simulink model "FinalCodev2_2"  (R2021b)
settings: Solver=ode23t  StartTime=0.0  StopTime=inf  RelTol=1e-3
InitFcn:
  | RPInit
model workspace (MAT data in the model file):
  mapForSim : object (value not decoded)
  occGrid : robotics.BinaryOccupancyGrid (value not decoded)
undefined symbols (not defined in the file or in its folder): X, Y, Z
libraries: sm_lib x25, nesl_utility x11, RP_Simulator_Components x7, ME598_ProjectLibrary x6, RoboticsPlayground x2, Contact_Forces_Lib x2
(part 2 of 2)

== stateflow chart FinalCodev2_2/Chart ==
  state DriveForward [commented out]
    LMotor = 100
    RMotor = 100
  state PivotRight [commented out]
    LMotor = -100
    RMotor = 100
  state GoToFirstPuck [commented out]
    state DriveForward1 [commented out]
      LeftM = 100;
      RightM = 100;
    state PivotLeft [commented out]
      entry, during:
      theta = atan2d(1.5-y,0-x);
      LeftM = -40;
      RightM = 40;
    state Stop [commented out]
      LeftM = 0;
      RightM = 0;
    (default) -> GoToFirstPuck.PivotLeft [commented out]
    GoToFirstPuck.PivotLeft -> GoToFirstPuck.DriveForward1 [commented out] : [t>theta-5 && t<theta+2]
    GoToFirstPuck.DriveForward1 -> GoToFirstPuck.Stop [commented out] : [Red_Distance < 0.42 && Red_Distance > 0.4]
  state GoToSecondPuck [commented out]
    state DriveForward1 [commented out]
      LeftM = 100;
      RightM = 100;
    state PivotRight [commented out]
      entry, during:
      theta = atan2d(-1.5-y,0-x);
      LeftM = 60;
      RightM = -60;
    state Stop [commented out]
      LeftM = 0;
      RightM = 0;
    (default) -> GoToSecondPuck.PivotRight [commented out]
    GoToSecondPuck.PivotRight -> GoToSecondPuck.DriveForward1 [commented out] : [t>theta-5 && t<theta+2]
    GoToSecondPuck.DriveForward1 -> GoToSecondPuck.Stop [commented out] : [Blue_Distance < 0.42 && Blue_Distance > 0.4]
  state NotCenter [commented out]
    LMotor = 100;
    RMotor = 100;
  state Centered [commented out]
    LMotor = 0;
    RMotor = 0;
  state GoToFirstPuck1
    state PivotLeft
      entry, during:
      theta = atan2d(1.5-y,0-x);
      LeftM = -15;
      RightM = 15;
    state DriveForward1
      entry,during:
      LeftM = 100;
      RightM = 100;
      exit:
      LeftM = 0;
      RightM = 0;
    (default) -> GoToFirstPuck1.PivotLeft
    GoToFirstPuck1.PivotLeft -> GoToFirstPuck1.DriveForward1 : [t>theta-2 && t<theta+2]
  note: NOTES:
      | - Consider a transition loop of pivotleft, pivotright, and moveforward for
      | each larger state blocks.
      | - If the puck is not completely centered on the manipulator, then it will
      | make the robot steer in the direction where the puck is leaning. For
      | example, if the puck is on the left side of the manipulator and you want
      | the robot to move forward, then it will slightly steer to the left. This is
      | unwanted behavior, so it is good to make sure that the theta pose of the
      | robot is always compared to the target pose so the robot doesn't stray from
      | the desired path.
      | - check the closest pivot!
  state GoToFirstEndzone [commented out]
    state PivotRight [commented out]
      entry,during:
      theta = atan2d(2.3-y, 2.3-x);
      LeftM = 40;
      RightM = -40;
    state DriveForward2 [commented out]
      LeftM = 80;
      RightM = 80;
    state Reverse [commented out]
      LeftM = -100;
      RightM = -100;
    state Stop2 [commented out]
      LeftM =0;
      RightM = 0;
    (default) -> GoToFirstEndzone.PivotRight [commented out]
    GoToFirstEndzone.PivotRight -> GoToFirstEndzone.DriveForward2 [commented out] : [t>theta-5 && t< theta+2]
    GoToFirstEndzone.DriveForward2 -> GoToFirstEndzone.Reverse [commented out] : [FrontSensor <0.7]
    GoToFirstEndzone.Reverse -> GoToFirstEndzone.Stop2 [commented out] : after(2,sec)
  state GoToSecondEndzone [commented out]
    state PivotRight [commented out]
      entry,during:
      theta = atan2d(0-y, -2.3-x);
      LeftM = 40;
      RightM = -40;
    state DriveForward2 [commented out]
      LeftM = 80;
      RightM = 80;
    state Reverse [commented out]
      LeftM = -100;
      RightM = -100;
    state Stop2 [commented out]
      LeftM =0;
      RightM = 0;
    (default) -> GoToSecondEndzone.PivotRight [commented out]
    GoToSecondEndzone.PivotRight -> GoToSecondEndzone.DriveForward2 [commented out] : [t>theta-5 && t< theta+2]
    GoToSecondEndzone.DriveForward2 -> GoToSecondEndzone.Reverse [commented out] : [FrontSensor <0.7]
    GoToSecondEndzone.Reverse -> GoToSecondEndzone.Stop2 [commented out] : after(2,sec)
  state GoToRedEndzone
    state PivotRight
      entry,during:
      theta = atan2d(2.2-y, 2.3-x);
      LeftM = 15;
      RightM = -15;
    state DriveForward2
      entry,during:
      theta = atan2d(2.2-y,2.3-x)
      LeftM = 80;
      RightM = 80;
    state Reverse
      entry,during:
      LeftM = -100;
      RightM = -100;
      exit:
      LeftM = 0;
      RightM = 0;
    state LeftWallAvoid
      entry,during:
      LeftM = 80;
      RightM = 0;
    state RightWallAvoid
      entry,during:
      LeftM = 0;
      RightM = 80;
    (default) -> GoToRedEndzone.PivotRight
    GoToRedEndzone.DriveForward2 -> GoToRedEndzone.PivotRight [order 2] : [(t-theta)>0]
    GoToRedEndzone.PivotRight -> GoToRedEndzone.DriveForward2 : [t>theta-2 && t< theta+2]
    GoToRedEndzone.DriveForward2 -> GoToRedEndzone.Reverse [order 1] : [FrontSensor <0.7]
    GoToRedEndzone.DriveForward2 -> GoToRedEndzone.LeftWallAvoid [order 3] : [LeftSensor <.01]
    GoToRedEndzone.LeftWallAvoid -> GoToRedEndzone.DriveForward2 : [LeftSensor >= .01]
    GoToRedEndzone.DriveForward2 -> GoToRedEndzone.RightWallAvoid [order 4] : [RightSensor<.01]
    GoToRedEndzone.RightWallAvoid -> GoToRedEndzone.DriveForward2 : [RightSensor>=.01]
  state GoToGreenEndzone
    state DriveForward2
      entry,during:
      theta = atan2d(-2.4-y, 2.2-x)
      LeftM = 80;
      RightM = 80;
    state PivotRight
      entry,during:
      theta = atan2d(-2.4-y, 2.2-x);
      LeftM = 15;
      RightM = -15;
    state Reverse
      entry,during:
      LeftM = -100;
      RightM = -100;
      exit:
      LeftM = 0;
      RightM = 0;
    state LeftWallAvoid
      entry,during:
      LeftM = 80;
      RightM = 0;
    state RightWallAvoid
      entry,during:
      LeftM = 0;
      RightM = 80;
    (default) -> GoToGreenEndzone.PivotRight
    GoToGreenEndzone.DriveForward2 -> GoToGreenEndzone.PivotRight [order 3] : [(t-theta) > 0]
    GoToGreenEndzone.PivotRight -> GoToGreenEndzone.DriveForward2 : [t>theta-2 && t< theta+2]
    GoToGreenEndzone.DriveForward2 -> GoToGreenEndzone.LeftWallAvoid [order 2] : [LeftSensor <.01]
    GoToGreenEndzone.LeftWallAvoid -> GoToGreenEndzone.DriveForward2 : [LeftSensor >= .01]
    GoToGreenEndzone.DriveForward2 -> GoToGreenEndzone.RightWallAvoid [order 4] : [RightSensor<.01]
    GoToGreenEndzone.RightWallAvoid -> GoToGreenEndzone.DriveForward2 : [RightSensor>=.01]
    GoToGreenEndzone.DriveForward2 -> GoToGreenEndzone.Reverse [order 1] : [FrontSensor <0.7]
  state GoToBlueEndzone
    state PivotRight
      entry,during:
      theta = atan2d(0-y, -2.3-x);
      LeftM = 15;
      RightM = -15;
    state DriveForward2
      entry,during:
      theta = atan2d(0-y,-2.3-x)
      LeftM = 80;
      RightM = 80;
    state Reverse
      entry,during:
      LeftM = -100;
      RightM = -100;
      exit:
      LeftM = 0;
      RightM = 0;
    state LeftWallAvoid
      entry,during:
      LeftM = 80;
      RightM = 0;
    state RightWallAvoid
      entry,during:
      LeftM = 0;
      RightM = 80;
    (default) -> GoToBlueEndzone.PivotRight
    GoToBlueEndzone.DriveForward2 -> GoToBlueEndzone.PivotRight [order 3] : [(t-theta) > 0]
    GoToBlueEndzone.PivotRight -> GoToBlueEndzone.DriveForward2 : [t>theta-2 && t< theta+2]
    GoToBlueEndzone.DriveForward2 -> GoToBlueEndzone.Reverse [order 1] : [FrontSensor <0.7]
    GoToBlueEndzone.DriveForward2 -> GoToBlueEndzone.LeftWallAvoid [order 2] : [LeftSensor <.01]
    GoToBlueEndzone.LeftWallAvoid -> GoToBlueEndzone.DriveForward2 : [LeftSensor >= .01]
    GoToBlueEndzone.DriveForward2 -> GoToBlueEndzone.RightWallAvoid [order 4] : [RightSensor<.01]
    GoToBlueEndzone.RightWallAvoid -> GoToBlueEndzone.DriveForward2 : [RightSensor>=.01]
  state GoToSecondPuck1
    state RightWallAvoid
      entry,during:
      LeftM = 0;
      RightM = 80;
    state DriveForward1
      entry,during:
      LeftM = 100;
      RightM = 100;
      exit:
      LeftM = 0;
      RightM = 0;
    state PivotLeft
      entry, during:
      theta = atan2d(-1.5-y,0-x);
      LeftM = -15;
      RightM = 15;
    state LeftWallAvoid
      entry,during:
      LeftM = 80;
      RightM = 0;
    GoToSecondPuck1.RightWallAvoid -> GoToSecondPuck1.DriveForward1 : [RightSensor>=.01]
    GoToSecondPuck1.DriveForward1 -> GoToSecondPuck1.RightWallAvoid [order 2] : [RightSensor<.01]
    (default) -> GoToSecondPuck1.PivotLeft
    GoToSecondPuck1.PivotLeft -> GoToSecondPuck1.DriveForward1 : [t>theta-2 && t<theta+2]
    GoToSecondPuck1.LeftWallAvoid -> GoToSecondPuck1.DriveForward1 : [LeftSensor >= .01]
    GoToSecondPuck1.DriveForward1 -> GoToSecondPuck1.LeftWallAvoid [order 3] : [LeftSensor <.01]
  state GoToRedEndzone1
    state PivotRight
      entry,during:
      theta = atan2d(2.1-y, 2.3-x);
      LeftM = 15;
      RightM = -15;
    state DriveForward2
      entry,during:
      theta = atan2d(2.1-y, 2.3-x)
      LeftM = 80;
      RightM = 80;
    state Reverse
      entry,during:
      LeftM = -100;
      RightM = -100;
      exit:
      LeftM = 0;
      RightM = 0;
    state LeftWallAvoid
      entry,during:
      LeftM = 80;
      RightM = 0;
    state RightWallAvoid
      entry,during:
      LeftM = 0;
      RightM = 80;
    (default) -> GoToRedEndzone1.PivotRight
    GoToRedEndzone1.DriveForward2 -> GoToRedEndzone1.PivotRight [order 4] : [(t-theta) > 0]
    GoToRedEndzone1.PivotRight -> GoToRedEndzone1.DriveForward2 : [t>theta-2 && t< theta+2]
    GoToRedEndzone1.DriveForward2 -> GoToRedEndzone1.Reverse [order 1] : [FrontSensor <0.7]
    GoToRedEndzone1.DriveForward2 -> GoToRedEndzone1.LeftWallAvoid [order 3] : [LeftSensor <.01]
    GoToRedEndzone1.LeftWallAvoid -> GoToRedEndzone1.DriveForward2 : [LeftSensor >= .01]
    GoToRedEndzone1.DriveForward2 -> GoToRedEndzone1.RightWallAvoid [order 2] : [RightSensor<.01]
    GoToRedEndzone1.RightWallAvoid -> GoToRedEndzone1.DriveForward2 : [RightSensor>=.01]
  state GoToGreenEndzone1
    state PivotRight
      entry,during:
      theta = atan2d(-2.1-y, 2.1-x);
      LeftM = 15;
      RightM = -15;
    state DriveForward
      LeftM = 80;
      RightM = 80;
    state Reverse
      entry,during:
      LeftM = -100;
      RightM = -100;
      exit:
      LeftM = 0;
      RightM = 0;
    state LeftWallAvoid
      entry,during:
      LeftM = 80;
      RightM = 0;
    state RightWallAvoid
      entry,during:
      LeftM = 0;
      RightM = 80;
    (default) -> GoToGreenEndzone1.PivotRight
    GoToGreenEndzone1.PivotRight -> GoToGreenEndzone1.DriveForward : [t>theta-2 && t< theta+2]
    GoToGreenEndzone1.DriveForward -> GoToGreenEndzone1.Reverse [order 1] : [FrontSensor <0.7]
    GoToGreenEndzone1.DriveForward -> GoToGreenEndzone1.LeftWallAvoid [order 3] : [LeftSensor <.01]
    GoToGreenEndzone1.LeftWallAvoid -> GoToGreenEndzone1.DriveForward : [LeftSensor >= .01]
    GoToGreenEndzone1.DriveForward -> GoToGreenEndzone1.RightWallAvoid [order 2] : [RightSensor<.01]
    GoToGreenEndzone1.RightWallAvoid -> GoToGreenEndzone1.DriveForward : [RightSensor>=.01]
  state GoToBlueEndzone1
    state PivotRight
      entry,during:
      theta = atan2d(0-y, -2.1-x);
      LeftM = 15;
      RightM = -15;
    state DriveForward
      entry,during:
      theta = atan2d(0-y,-2.1-x)
      LeftM = 80;
      RightM = 80;
    state Reverse
      entry,during:
      LeftM = -100;
      RightM = -100;
      exit:
      LeftM = 0;
      RightM = 0;
    state LeftWallAvoid
      entry,during:
      LeftM = 80;
      RightM = 0;
    state RightWallAvoid
      entry,during:
      LeftM = 0;
      RightM = 80;
    (default) -> GoToBlueEndzone1.PivotRight
    GoToBlueEndzone1.DriveForward -> GoToBlueEndzone1.PivotRight [order 4] : [(t-theta) > 0]
    GoToBlueEndzone1.PivotRight -> GoToBlueEndzone1.DriveForward : [t>theta-2 && t< theta+2]
    GoToBlueEndzone1.DriveForward -> GoToBlueEndzone1.Reverse [order 1] : [FrontSensor <0.7]
    GoToBlueEndzone1.DriveForward -> GoToBlueEndzone1.LeftWallAvoid [order 3] : [LeftSensor <.01]
    GoToBlueEndzone1.LeftWallAvoid -> GoToBlueEndzone1.DriveForward : [LeftSensor >= .01]
    GoToBlueEndzone1.DriveForward -> GoToBlueEndzone1.RightWallAvoid [order 2] : [RightSensor<.01]
    GoToBlueEndzone1.RightWallAvoid -> GoToBlueEndzone1.DriveForward : [RightSensor>=.01]
  state gohome1
    state PivotLeft1
      entry, during:
      theta = atan2d(0-y,0-x);
      LeftM = -50;
      RightM = 50;
      exit:
      LeftM=0;
      RightM = 0;
    state diff_less
      entry,during:
      inv_diff = diff +360;
      abs1 = abs(diff)
    state DriveForward
      entry:
      after(0.2,sec)
      during:
      LeftM = 80;
      RightM = 80;
      theta = atan2d(0-y,0-x)
    state Reverse
      entry, during:
      LeftM = -60;
      RightM = -60;
      theta = atan2d(0-y,0-x)
      diff = t-theta
    state PivotRight
      entry, during:
      theta = atan2d(0-y,0-x);
      LeftM = 50;
      RightM = -50;
      exit:
      LeftM = 0;
      RightM = 0;
    state diff_great
      entry,during:
      inv_diff = diff -360;
      abs1 = abs(inv_diff)
    state Stop
      LeftM = 0;
      RightM = 0;
    PivotLeft1 -> gohome1.DriveForward : [t>theta-3.5 && t<theta+3.5]
    (default) -> gohome1.Reverse
    diff_less -> PivotLeft1 [order 1] : [inv_diff > abs1]
    gohome1.DriveForward -> PivotLeft1 [order 3] : [(t-(theta-3.5)) < 0]
    diff_great -> PivotLeft1 [order 1] : [diff > abs1]
    gohome1.Reverse -> diff_less [order 2] : [diff < 0]
    diff_less -> gohome1.PivotRight [order 2] : [inv_diff < abs1]
    gohome1.DriveForward -> gohome1.Stop [order 1] : [x > -0.2 && x < 0.2 && y > -0.2 && y < 0.2]
    gohome1.PivotRight -> gohome1.DriveForward : [t > theta -3.5 && t< theta +3.5]
    gohome1.DriveForward -> gohome1.PivotRight [order 2] : [(t-(theta+3.5)) > 0]
    gohome1.Reverse -> diff_great [order 1] : [diff > 0]
    diff_great -> gohome1.PivotRight [order 2] : [diff < abs1]
  (default) -> PivotRight [commented out]
  PivotRight -> DriveForward [commented out] : [Red_Distance >0]
  (default) -> GoToFirstPuck [commented out]
  DriveForward -> PivotRight [commented out] : [Red_Distance < 0]
  (default) -> NotCenter [commented out]
  NotCenter -> Centered [commented out] : [XPos>-0.05 && XPos <0.05]
  GoToFirstEndzone -> GoToSecondPuck [commented out] : after(1,sec)
  Centered -> NotCenter [commented out] : [XPos<-0.05 && XPos >0.05]
  (default) -> GoToFirstPuck1
  GoToFirstPuck.Stop -> GoToFirstEndzone [commented out] : after (1,sec)
  GoToSecondPuck.Stop -> GoToSecondEndzone [commented out] : after (1,sec)
  GoToFirstPuck1.DriveForward1 -> (junction 120) : [(Red_Distance < 0.42 && Red_Distance > 0.3) || (Green_Distance < 0.42 && Green_Distance > 0.3) || (Blue_Distance < 0.42 && Blue_Distance > 0.3)]
  (junction 120) -> GoToRedEndzone [order 1] : [Red_Distance > 0]
  (junction 120) -> GoToBlueEndzone [order 3] : [Blue_Distance >0]
  (junction 120) -> GoToGreenEndzone [order 2] : [Green_Distance > 0]
  GoToRedEndzone.Reverse -> (junction 152) : after(2,sec)
  GoToGreenEndzone.Reverse -> (junction 152) : after(2,sec)
  GoToBlueEndzone.Reverse -> (junction 152) : after (2,sec)
  (junction 152) -> GoToSecondPuck1 : after(2,sec)
  GoToSecondPuck1.DriveForward1 -> (junction 164) [order 1] : [(Red_Distance < 0.42 && Red_Distance > 0.3) || (Green_Distance < 0.42 && Green_Distance > 0.3) || (Blue_Distance < 0.42 && Blue_Distance > 0.3)]
  (junction 164) -> GoToRedEndzone1 [order 1] : [Red_Distance > 0]
  (junction 164) -> GoToBlueEndzone1 [order 3] : [Blue_Distance >0]
  (junction 164) -> GoToGreenEndzone1 [order 2] : [Green_Distance > 0]
  GoToRedEndzone1.Reverse -> (junction 192) : after(2,sec)
  GoToGreenEndzone1.Reverse -> (junction 192) : after(2,sec)
  GoToBlueEndzone1.Reverse -> (junction 192) : after (2,sec)
  (junction 192) -> gohome1 : after (9,sec)
  data: LeftM output; theta output; RightM output; x input; Red_Distance input; Green_Distance input; Blue_Distance input; y input; t input; FrontSensor input; LeftSensor input; RightSensor input; abs1 local; diff local; inv_diff local

== matlab function FinalCodev2_2/-180* : 180* ==
  data: deg input; deg output
function deg = degWrap(deg)

% % Convert radians to degrees
% deg = 180/pi * rad;


% Wrap degree value to the range -180* : +180*
for idx = 1:length(deg)
    while deg(idx) < -180
        deg(idx) = deg(idx)+360;
    end
    
    while deg(idx) > 180
        deg(idx) = deg(idx)-360;
    end
end

return

== matlab function FinalCodev2_2/-180* : 180*1 ==
  data: deg input; deg output
function deg = degWrap(deg)

% % Convert radians to degrees
% deg = 180/pi * rad;


% Wrap degree value to the range -180* : +180*
for idx = 1:length(deg)
    while deg(idx) < -180
        deg(idx) = deg(idx)+360;
    end
    
    while deg(idx) > 180
        deg(idx) = deg(idx)-360;
    end
end

return
